simulink model "Rocket_sim"  (R2021a)
settings: Solver=VariableStepAuto  StartTime=0.0  StopTime=180  FixedStep=0.1  RelTol=1e-3
libraries: simulink x3, shared3dof x1
settings Model: Creator=jk111  LastModifiedBy=jk111

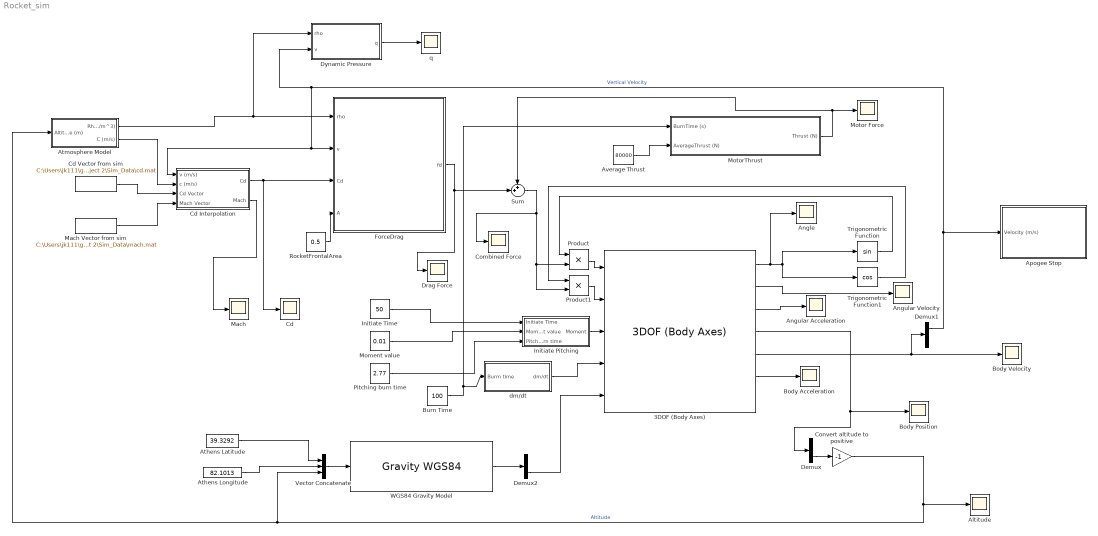
== system Rocket_sim ==
  3DOF (Body Axes) : shared3dof/3DOF (Body Axes)  units=Metric (MKS)  mtype=Simple Variable  v_ini=0  theta_ini=3.14159265359/2  alpha_ini=0  pos_ini=[0 0]  q_ini=0  mass=1446.58165  mass_e=111  mass_f=1447  Iyy=1.0  Iyy_e=0.5  Iyy_f=3.0  g_in=External  g=9.81  vre_flag=off  abi_flag=off  aMode=0  vel_statename=''  theta_statename=''  pos_statename=''  q_statename=''  mass_statename=''
      settings: SourceProductBaseCode=AE,PW,DR,MT,UV,VE
  Altitude : Scope
  Angle : Scope
  Angular Acceleration : Scope
  Angular Velocity : Scope
  Apogee Stop : Subsystem
  Athens Latitude : Constant  Value=39.3292
  Athens Longitude : Constant  Value=82.1013
  Atmosphere Model : Subsystem
  Average Thrust : Constant  Value=80000
  Body Acceleration : Scope
  Body Position : Scope
  Body Velocity : Scope
  Burn Time : Constant  Value=100
  Cd : Scope
  Cd Interpolation : Subsystem
  Cd Vector from sim : FromFile  FileName=C:\Users\jk111\github\ME6900_Rockets\Project 2\Sim_Data\cd.mat  SampleTime=0
  Combined Force : Scope
  Convert altitude to positive : Gain  Gain=-1
  Demux : Demux  Outputs=2
  Demux1 : Demux  Outputs=2
  Demux2 : Demux  Outputs=3
  Drag Force : Scope
  Dynamic Pressure : MATLAB Function  TreatAsAtomicUnit=on
  ForceDrag : MATLAB Function  TreatAsAtomicUnit=on
  Initiate Pitching : Subsystem
  Initiate Time : Constant  Value=50
  Mach : Scope
  Mach Vector from sim : FromFile  FileName=C:\Users\jk111\github\ME6900_Rockets\Project 2\Sim_Data\mach.mat  SampleTime=0
  Moment value : Constant  Value=0.01
  Motor Force : Scope
  MotorThrust : Subsystem
  Pitching burn time : Constant  Value=2.77
  Product : Product
  Product1 : Product
  RocketFrontalArea : Constant  Value=0.5
  Sum : Sum  Inputs=++|
  Trigonometric Function : Trigonometry
  Trigonometric Function1 : Trigonometry  Operator=cos
  Vector Concatenate : Concatenate  NumInputs=3
  "WGS84 Gravity Model  " : GravityWGS84  month=February  day=19  year=2024
  dm/dt : Subsystem
  q : Scope
  wires:
  RocketFrontalArea/1 -> ForceDrag/4(A)
  ForceDrag/1(fd) -> Sum/2, Drag Force/1
  MotorThrust/1(Thrust (N)) -> Sum/1, Motor Force/1
  3DOF (Body Axes)/5 -> Demux1/1, Body Velocity/1
  Demux1/1 -> Cd Interpolation/1(v (m/s)), ForceDrag/2(v), Dynamic Pressure/2(v), Apogee Stop/1(Velocity (m/s))  "Vertical Velocity"
  Demux/2 -> Convert altitude to positive/1
  Cd Interpolation/1(Cd) -> ForceDrag/3(Cd), Cd/1
  Vector Concatenate/1 -> "WGS84 Gravity Model  "/1
  Athens Longitude/1 -> Vector Concatenate/2
  Athens Latitude/1 -> Vector Concatenate/1
  "WGS84 Gravity Model  "/1 -> Demux2/1
  Demux2/3 -> 3DOF (Body Axes)/5
  Convert altitude to positive/1 -> Vector Concatenate/3, Atmosphere Model/1(Altitude (m)), Altitude/1  "Altitude"
  Cd Vector from sim/1 -> Cd Interpolation/3(Cd Vector)
  Mach Vector from sim/1 -> Cd Interpolation/4(Mach Vector)
  Average Thrust/1 -> MotorThrust/2(AverageThrust (N))
  3DOF (Body Axes)/6 -> Body Acceleration/1
  Dynamic Pressure/1(q) -> q/1
  Cd Interpolation/2(Mach) -> Mach/1
  Atmosphere Model/2(C (m/s)) -> Cd Interpolation/2(c (m/s))
  Atmosphere Model/1(Rho (kg/m^3)) -> Dynamic Pressure/1(rho), ForceDrag/1(rho)
  3DOF (Body Axes)/4 -> Demux/1, Body Position/1
  3DOF (Body Axes)/1 -> Angle/1, Trigonometric Function1/1, Trigonometric Function/1
  Product/1 -> 3DOF (Body Axes)/1
  Product1/1 -> 3DOF (Body Axes)/2
  Trigonometric Function/1 -> Product/1
  Trigonometric Function1/1 -> Product1/1
  Sum/1 -> Combined Force/1, Product1/2, Product/2
  Initiate Pitching/1(Moment) -> 3DOF (Body Axes)/3
  dm/dt/1(dm/dt) -> 3DOF (Body Axes)/4
  Moment value/1 -> Initiate Pitching/2(Moment value)
  Initiate Time/1 -> Initiate Pitching/1(Initiate Time)
  Pitching burn time/1 -> Initiate Pitching/3(Pitch burn time)
  Burn Time/1 -> MotorThrust/1(BurnTime (s)), dm/dt/1(Burm time)
  3DOF (Body Axes)/2 -> Angular Velocity/1
  3DOF (Body Axes)/3 -> Angular Acceleration/1

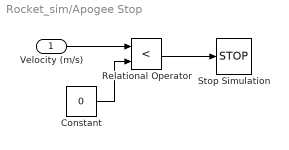
== system Rocket_sim/Apogee Stop ==
  Velocity (m/s) : Inport
  Constant : Constant  Value=0
  Relational Operator : RelationalOperator  Operator=<  OutDataTypeStr=boolean  RndMeth=Simplest
  Stop Simulation : Stop
  wires:
  Velocity (m/s)/1 -> Relational Operator/1
  Constant/1 -> Relational Operator/2
  Relational Operator/1 -> Stop Simulation/1

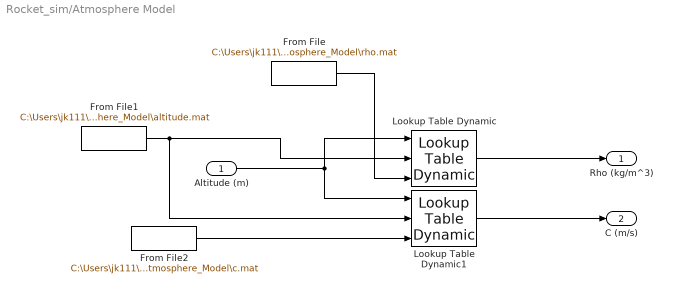
== system Rocket_sim/Atmosphere Model ==
  Altitude (m) : Inport
  From File : FromFile  FileName=C:\Users\jk111\github\ME6900_Rockets\Project 2\Atmosphere_Model\rho.mat  SampleTime=0
  From File1 : FromFile  FileName=C:\Users\jk111\github\ME6900_Rockets\Project 2\Atmosphere_Model\altitude.mat  SampleTime=0
  From File2 : FromFile  FileName=C:\Users\jk111\github\ME6900_Rockets\Project 2\Atmosphere_Model\c.mat  SampleTime=0
  Lookup Table Dynamic : simulink/Lookup Tables/Lookup Table Dynamic  LookUpMeth=Interpolation-Use End Values  OutDataType=fixdt('double')  OutScaling=[]  OutputDataTypeScalingMode=Specify via dialog  OutDataTypeStr=double  DoSatur=off
  Lookup Table Dynamic1 : simulink/Lookup Tables/Lookup Table Dynamic  LookUpMeth=Interpolation-Use End Values  OutDataType=fixdt('double')  OutScaling=[]  OutputDataTypeScalingMode=Specify via dialog  OutDataTypeStr=double  DoSatur=off
  Rho (kg/m^3) : Outport
  C (m/s) : Outport  Port=2
  wires:
  Lookup Table Dynamic1/1 -> C (m/s)/1
  Lookup Table Dynamic/1 -> Rho (kg/m^3)/1
  Altitude (m)/1 -> Lookup Table Dynamic1/1, Lookup Table Dynamic/1
  From File2/1 -> Lookup Table Dynamic1/3
  From File/1 -> Lookup Table Dynamic/3
  From File1/1 -> Lookup Table Dynamic1/2, Lookup Table Dynamic/2

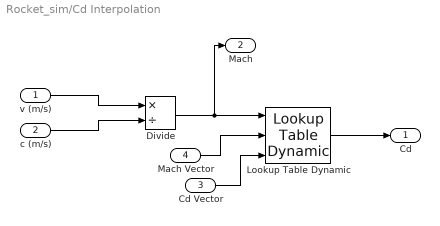
== system Rocket_sim/Cd Interpolation ==
  v (m/s) : Inport
  c (m/s) : Inport  Port=2
  Cd Vector : Inport  Port=3
  Mach Vector : Inport  Port=4
  Divide : Product  Inputs=*/
  Lookup Table Dynamic : simulink/Lookup Tables/Lookup Table Dynamic  LookUpMeth=Use Input Nearest  OutDataType=fixdt('double')  OutScaling=[]  OutputDataTypeScalingMode=Specify via dialog  OutDataTypeStr=double  DoSatur=off
  Cd : Outport
  Mach : Outport  Port=2
  wires:
  Lookup Table Dynamic/1 -> Cd/1
  c (m/s)/1 -> Divide/2
  v (m/s)/1 -> Divide/1
  Divide/1 -> Mach/1, Lookup Table Dynamic/1
  Cd Vector/1 -> Lookup Table Dynamic/3
  Mach Vector/1 -> Lookup Table Dynamic/2

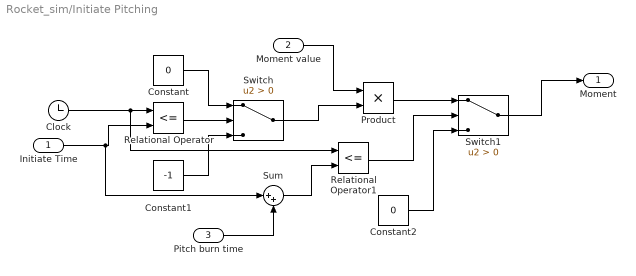
== system Rocket_sim/Initiate Pitching ==
  Initiate Time : Inport
  Moment value : Inport  Port=2
  Pitch burn time : Inport  Port=3
  Clock : Clock
  Constant : Constant  Value=0
  Constant1 : Constant  Value=-1
  Constant2 : Constant  Value=0
  Product : Product
  Relational Operator : RelationalOperator  Operator=<=  OutDataTypeStr=boolean  RndMeth=Simplest
  Relational Operator1 : RelationalOperator  Operator=<=  OutDataTypeStr=boolean  RndMeth=Simplest
  Sum : Sum  Inputs=|++
  Switch : Switch  Criteria=u2 > Threshold
  Switch1 : Switch  Criteria=u2 > Threshold
  Moment : Outport
  wires:
  Relational Operator/1 -> Switch/2
  Constant/1 -> Switch/1
  Constant1/1 -> Switch/3
  Initiate Time/1 -> Sum/1, Relational Operator/2
  Clock/1 -> Relational Operator1/1, Relational Operator/1
  Switch/1 -> Product/2
  Moment value/1 -> Product/1
  Product/1 -> Switch1/1
  Switch1/1 -> Moment/1
  Constant2/1 -> Switch1/3
  Relational Operator1/1 -> Switch1/2
  Pitch burn time/1 -> Sum/2
  Sum/1 -> Relational Operator1/2

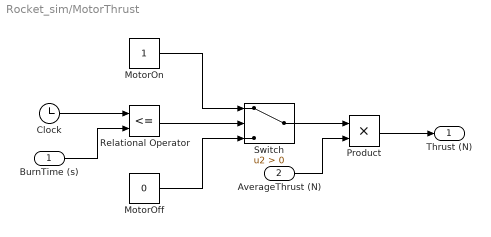
== system Rocket_sim/MotorThrust ==
  BurnTime (s) : Inport
  AverageThrust (N) : Inport  Port=2
  Clock : Clock
  MotorOff : Constant  Value=0
  MotorOn : Constant
  Product : Product
  Relational Operator : RelationalOperator  Operator=<=  OutDataTypeStr=boolean  RndMeth=Simplest
  Switch : Switch  Criteria=u2 > Threshold
  Thrust (N) : Outport
  wires:
  MotorOn/1 -> Switch/1
  MotorOff/1 -> Switch/3
  Relational Operator/1 -> Switch/2
  Clock/1 -> Relational Operator/1
  BurnTime (s)/1 -> Relational Operator/2
  Switch/1 -> Product/1
  AverageThrust (N)/1 -> Product/2
  Product/1 -> Thrust (N)/1

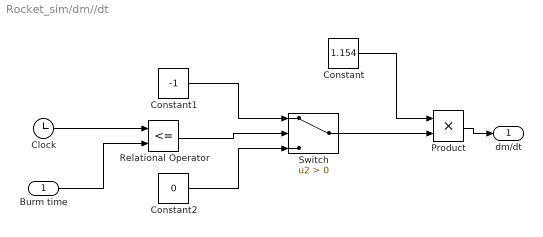
== system Rocket_sim/dm//dt ==
  Burm time : Inport
  Clock : Clock
  Constant : Constant  Value=1.154
  Constant1 : Constant  Value=-1
  Constant2 : Constant  Value=0
  Product : Product
  Relational Operator : RelationalOperator  Operator=<=  OutDataTypeStr=boolean  RndMeth=Simplest
  Switch : Switch  Criteria=u2 > Threshold
  dm/dt : Outport
  wires:
  Product/1 -> dm/dt/1
  Constant/1 -> Product/1
  Switch/1 -> Product/2
  Constant1/1 -> Switch/1
  Constant2/1 -> Switch/3
  Relational Operator/1 -> Switch/2
  Burm time/1 -> Relational Operator/2
  Clock/1 -> Relational Operator/1

== matlab function Rocket_sim/Dynamic Pressure ==
  data: rho input; q output; v input
function q = DynamicPressure(rho, v)

q = (1/2)*rho*v^2;

== matlab function Rocket_sim/ForceDrag ==
  data: rho input; fd output; v input; Cd input; A input
function fd = drag(rho,v,Cd,A)

fd = (-1/2)*rho*v^2*Cd*A;
